simulink model "SMIB_test_SL_2023a_Copy"  (R2023a)
settings: Solver=FixedStepAuto  StartTime=0.0  StopTime=30.0  FixedStep=1e-4  RelTol=1e-3
undefined symbols (not defined in the file or in its folder): Angle, D1, Delta, Magnitude
libraries: spsThreePhaseSeriesRLCLoadLib x4, spsThreePhasePISectionLineLib x2, spsThreePhaseBreakerLib x2, ee_lib x1, spsExcitationSystemLib x1, spsHydraulicTurbineandGovernorLib x1, spsSynchronousMachinepuFundamentalLib x1, spsThreePhaseDynamicLoadLib x1, spsThreePhaseTransformerTwoWindingsLib x1, spsThreePhaseVIMeasurementLib x1, spsThreePhaseFaultLib x1, spsThreePhaseSourceLib x1
settings Model: Creator=shaohui  LastModifiedBy=lab-admin

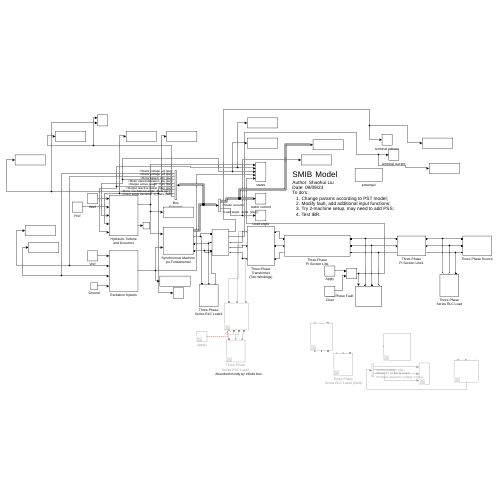
[thumbnail: Simulink's stored preview of the top-level diagram]
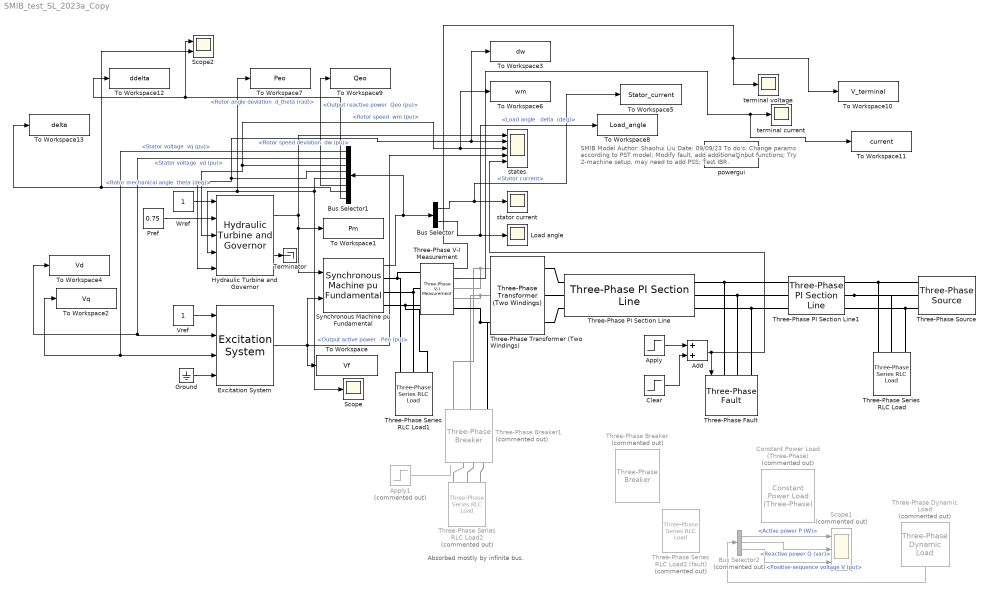
== system SMIB_test_SL_2023a_Copy ==
  note: Absorbed mostly by infinite bus.
  note: SMIB Model
      | Author: Shaohui Liu
      | Date: 09/09/23
      | To do's:
      | Change params according to PST model;
      | Modify fault, add additional input functions;
      | Try 2-machine setup, may need to add PSS;
      | Test IBR.
  Add : Sum
  Apply : Step  Time=15  After=5  SampleTime=0
  Apply1 : Step  Commented=on  Time=23  SampleTime=0
  Bus Selector : BusSelector  OutputSignals="Stator current,Load angle   delta  (deg)"
  Bus Selector1 : BusSelector  OutputSignals="dq0 components.Stator voltage  vq (pu),dq0 components.Stator voltage  vd (pu),Mechanical.Rotor speed  wm (pu),Mechanical.Rotor speed deviation  dw (pu),Output active power   Peo (pu),Output reactive power  Qeo (pu),Mechanical.Rotor mechanical angle  theta (deg),Mechanical.Rotor angle deviation  d_theta (rad)"
  Bus Selector2 : BusSelector  Commented=on  OutputSignals=Active power P (W),Reactive power Q (var),Positive-sequence voltage V (pu)
  Clear : Step  Time=15.1667  After=-5  SampleTime=0
  Constant Power Load (Three-Phase) : ee_lib/Passive/Constant Power Load (Three-Phase)  Commented=on  port_option=ee.enum.threePhasePort.composite  FRated=60 Hz  active_power=1 kW  reactive_power=0 A*kV  Vline_rms_min=100 V  tau=0.01 s  Vline_rms_ini=200 V  Vang_ini=0 deg  gmin=1e-6 S  enable_fault=simscape.enum.onoff.off  fault_action=simscape.enum.assert.action.none  t_fault=1 s  open_conductance=1e-4 S
      settings: InternalSimscapePortConfiguration="{\"Bottom\":[],\"Left\":[{\"id\":\"N\",\"label\":\"~\",\"type\":\"foundation.electrical.three_phase\"}],\"Right\":[],\"Top\":[]}"
  Excitation System : spsExcitationSystemLib/Excitation System  tr=20e-3  reg=[ 300, 0.001 ]  exc=[ 1, 0 ]  tgr=[ 0, 0 ]  damp=[ 0.001, 0.1 ]  sat=[ 0, 0 ]  lim=[ -11.5, 11.5, 0 ]  v0="[1.0  1.28]"
      settings: LibrarySourceBlock=sps_lib/Electrical Machines/Synchronous Machine Control/Excitation System
  Ground : Ground
  Hydraulic Turbine and Governor : spsHydraulicTurbineandGovernorLib/Hydraulic Turbine and Governor  sm="[ 10/3  0.07 ]"  gate="[  0.01  0.97518  -0.1  0.1 ]"  reg="[  0.05  1.163  0.105  0  0.01  ]"  hyd="[  0  2.67  ]"  dref=0  po=0.7516
      settings: LibrarySourceBlock=|
      | sps_lib/Electrical Machines/Synchronous Machine Control/Hydraulic Turbine
      | and Governor
  Load angle : Scope
  Pref : Constant  Value=0.75
  Scope : Scope
  Scope1 : Scope  Commented=on  NumInputPorts=3
  Scope2 : Scope  NumInputPorts=2
  Synchronous Machine pu Fundamental : spsSynchronousMachinepuFundamentalLib/Synchronous Machine pu Fundamental  PresetModel=No  MechanicalLoad=Mechanical power Pm  ShowDetailedParameters=on  RotorType=Salient-pole  Units=per unit fundamental parameters  MeasurementBus=off  NominalParameters="[ 187E6  13800   60]"  Stator="[ 2.85E-03  0.114  1.19  0.36 ]"  Field="[ 5.79E-04  0.114]"  Dampers2=[0.0652, 0.5134, 0.0287, 0.2553, 7.765e-3, 0.9167 ]  Dampers1="[ 1.17E-02  0.182  1.97E-02  0.384 ]"  Mechanical=[ 3.7 0 20]  PolePairs=20  InitialConditions="[ 0  0  0  0  0  0  0  0  1 ]"  SetSaturation=off  Saturation=[0.6404,0.7127,0.8441,0.9214,0.9956,1.082,1.19,1.316,1.457;0.7,0.7698,0.8872,0.9466,0.9969,1.046,1.1,1.151,1.201]  LoadFlowParameters=[1,0,0,0,0]  TsPowergui=0  TsBlock=-1  IterativeModel=Trapezoidal non iterative  IterativeDiscreteModel=Trapezoidal non iterative  BusType=PV  Pref=0  Qref=0  Qmin=-inf  Qmax=inf  PLF=0  QLF=0
      settings: LibrarySourceBlock=|
      | sps_lib/Electrical Machines/Synchronous Machine
      | pu Fundamental
  Terminator : Terminator
  Three-Phase Dynamic Load : spsThreePhaseDynamicLoadLib/Three-Phase Dynamic Load  Commented=on  NominalVoltage=[ 13.8e3 60 ]  ActiveReactivePowers=[50e6 25e6]  PositiveSequence=[0.994 -11.8]  ExternalControl=off  NpNq=[1.3 2]  TimeConstants="[0  0  0  0]"  MinimumVoltage=0.7  Tfilter=1e-4  LoadFlowParameters=[4,0,0,0,0]
      settings: LibrarySourceBlock=|
      | sps_lib/Passives/Three-Phase
      | Dynamic Load
  Three-Phase PI Section Line : spsThreePhasePISectionLineLib/Three-Phase PI Section Line  LConnTagsString=a|b|c  RConnTagsString=A|B|C  Length=95  Frequency=60  Resistances=[ 0.01273 0.3864]  Inductances="[ 0.9337e-3  4.1264e-3]"  Capacitances=[12.74e-9 7.751e-9]
  Three-Phase PI Section Line1 : spsThreePhasePISectionLineLib/Three-Phase PI Section Line  LConnTagsString=a|b|c  RConnTagsString=A|B|C  Length=5  Frequency=60  Resistances=[ 0.01273 0.3864]  Inductances="[ 0.9337e-3  4.1264e-3]"  Capacitances=[12.74e-9 7.751e-9]
  Three-Phase Series RLC Load : spsThreePhaseSeriesRLCLoadLib/Three-Phase Series RLC Load  LConnTagsString=A|B|C  Configuration=Y (grounded)  NominalVoltage=230e3  Vabc=[1e3 1e3 1e3]  Vabcp=[1e3 1e3 1e3]  NominalFrequency=60  UnbalancedPower=off  ActivePower=10e3  InductivePower=100  CapacitivePower=100  Pabc=[10e3 9e3 11e3]  QLabc=[100 90 110]  QCabc=[100 90 110]  Pabcp=[10e3 9e3 11e3]  QLabcp=[100 90 110]  QCabcp=[100 90 110]  Measurements=None  LoadType=constant Z
  Three-Phase Series RLC Load1 : spsThreePhaseSeriesRLCLoadLib/Three-Phase Series RLC Load  LConnTagsString=A|B|C  Configuration=Y (grounded)  NominalVoltage=13.8e3  Vabc=[1e3 1e3 1e3]  Vabcp=[1e3 1e3 1e3]  NominalFrequency=60  UnbalancedPower=off  ActivePower=10e3  InductivePower=0  CapacitivePower=0  Pabc=[10e3 9e3 11e3]  QLabc=[100 90 110]  QCabc=[100 90 110]  Pabcp=[10e3 9e3 11e3]  QLabcp=[100 90 110]  QCabcp=[100 90 110]  Measurements=None  LoadType=constant Z
  Three-Phase Series RLC Load2 : spsThreePhaseSeriesRLCLoadLib/Three-Phase Series RLC Load  Commented=on  LConnTagsString=A|B|C  Configuration=Y (grounded)  NominalVoltage=13.8e3  Vabc=[13.8e3 13.8e3 13.8e3]  Vabcp=[13.8e3 13.8e3 13.8e3]  NominalFrequency=60  UnbalancedPower=on  ActivePower=100e3  InductivePower=0  CapacitivePower=0  Pabc=[10000e3 10000e3 10000e3]  QLabc=[1000 1000 1000]  QCabc=[1000 1000 1000]  Pabcp=[1000e3 900e3 1100e3]  QLabcp=[100 90 110]  QCabcp=[100 90 110]  Measurements=None  LoadType=constant PQ
  Three-Phase Series RLC Load2 (fault) : spsThreePhaseSeriesRLCLoadLib/Three-Phase Series RLC Load  Commented=on  LConnTagsString=A|B|C  Configuration=Y (grounded)  NominalVoltage=13.8e3  Vabc=[1e3 1e3 1e3]  Vabcp=[1e3 1e3 1e3]  NominalFrequency=60  UnbalancedPower=off  ActivePower=100e3  InductivePower=100  CapacitivePower=100  Pabc=[10e3 9e3 11e3]  QLabc=[100 90 110]  QCabc=[100 90 110]  Pabcp=[10e3 9e3 11e3]  QLabcp=[100 90 110]  QCabcp=[100 90 110]  Measurements=Branch voltages and currents  LoadType=constant Z
  Three-Phase Transformer (Two Windings) : spsThreePhaseTransformerTwoWindingsLib/Three-Phase Transformer (Two Windings)  Winding1Connection=Delta (D1)  Winding2Connection=Yg  CoreType=Three single-phase transformers  SetSaturation=off  Hysteresis=off  DataFile='hysteresis'  SetInitialFlux=off  Measurements=None  UNITS=pu  NominalPower=[ 250e6 , 60 ]  Winding1=[13.8e3 , 0.002 , 0.08 ]  Winding2=[ 230e3 , 0.002 , 0.08 ]  Rm=500  Lm=500  L0=0.5  Saturation=[ 0,0 ; 0.0024,1.2 ; 1.0,1.52 ]  InitialFluxes=[ 0.8 , -0.8 , 0.7 ]  BreakLoop=off  DiscreteSolver=Trapezoidal iterative  DataType=off  TransfoNumber=1
  Three-Phase V-I Measurement : spsThreePhaseVIMeasurementLib/Three-Phase V-I Measurement  VoltageMeasurement=phase-to-phase  SetLabelV=off  LabelV=Vabc  Vpu=off  VpuLL=off  CurrentMeasurement=yes  SetLabelI=off  LabelI=Iabc  Ipu=off  Pbase=100e6  Vbase=500e3  OutputType=Magnitude-Angle  PhasorSimulation=on  PSBequivalent=0
  Three-Phase Breaker : spsThreePhaseBreakerLib/Three-Phase Breaker  Commented=on  InitialState=closed  SwitchA=on  SwitchB=on  SwitchC=on  SwitchTimes="[20.5  20.5+5/60]"  External=off  BreakerResistance=0.01  SnubberResistance=1e6  SnubberCapacitance=inf  Measurements=Breaker voltages and currents
  Three-Phase Breaker1 : spsThreePhaseBreakerLib/Three-Phase Breaker  Commented=on  InitialState=open  SwitchA=on  SwitchB=on  SwitchC=on  SwitchTimes="[23  23+30/60]"  External=on  BreakerResistance=0.01  SnubberResistance=1e6  SnubberCapacitance=inf  Measurements=None
  Three-Phase Fault : spsThreePhaseFaultLib/Three-Phase Fault  InitialStates=0  FaultA=on  FaultB=on  FaultC=on  GroundFault=on  SwitchTimes="[15  15+2/60]"  External=on  SwitchStatus=NaN  FaultResistance=0.001  GroundResistance=0.01  SnubberResistance=1e6  SnubberCapacitance=inf  Measurements=Fault voltages and currents
  Three-Phase Source : spsThreePhaseSourceLib/Three-Phase Source  InternalConnection=Yg  VoltagePhases=off  Voltage=230e3  PhaseAngle=0  Voltage_phases=[25e3 25e3 25e3]/sqrt(3)  PhaseAngles_phases=[0 -120 +120]  Frequency=60  NonIdealSource=on  SpecifyImpedance=off  Resistance=0.8929  Inductance=16.58e-3  ShortCircuitLevel=100e6  BaseVoltage=25e3  XRratio=7  BusType=swing  Pref=10e3  Qref=0  Prefabc=[10e3, 10e3, 10e3]  Qrefabc=[0, 0, 0]  Qmin=-inf  Qmax=inf
  To Workspace : ToWorkspace  VariableName=Vf  SaveFormat=Timeseries  SampleTime=-1
  To Workspace1 : ToWorkspace  VariableName=Pm  SaveFormat=Timeseries  SampleTime=-1
  To Workspace10 : ToWorkspace  VariableName=V_terminal  SaveFormat=Timeseries  SampleTime=-1
  To Workspace11 : ToWorkspace  VariableName=current  SaveFormat=Timeseries  SampleTime=-1
  To Workspace12 : ToWorkspace  VariableName=ddelta  SaveFormat=Timeseries  SampleTime=-1
  To Workspace13 : ToWorkspace  VariableName=delta  SaveFormat=Timeseries  SampleTime=-1
  To Workspace2 : ToWorkspace  VariableName=Vq  SaveFormat=Timeseries  SampleTime=-1
  To Workspace3 : ToWorkspace  VariableName=dw  SaveFormat=Timeseries  SampleTime=-1
  To Workspace4 : ToWorkspace  VariableName=Vd  SaveFormat=Timeseries  SampleTime=-1
  To Workspace5 : ToWorkspace  VariableName=Stator_current  SaveFormat=Timeseries  SampleTime=-1
  To Workspace6 : ToWorkspace  VariableName=wm  SaveFormat=Timeseries  SampleTime=-1
  To Workspace7 : ToWorkspace  VariableName=Peo  SaveFormat=Timeseries  SampleTime=-1
  To Workspace8 : ToWorkspace  VariableName=Load_angle  SaveFormat=Timeseries  SampleTime=-1
  To Workspace9 : ToWorkspace  VariableName=Qeo  SaveFormat=Timeseries  SampleTime=-1
  Vref : Constant
  Wref : Constant
  powergui : sps_lib/powergui  Priority=1  SimulationMode=Phasor  SampleTime=50e-6  frequency=60  Iterations=50  frequencyindice=60  Pbase=100e6  ErrMax=1e-4  UnitsV=kV  UnitsW=MW  buscounter=0  FunctionMessages=off  echomessages=off  EnableUseOfTLC=off  CurrentSourceSwitches=off  DisableSnubberDevices=off  DisableRonSwitches=off  DisableVfSwitches=off  DisplayEquations=off  AutomaticDiscreteSolvers=off  SolverType=Tustin/Backward Euler (TBE)  Interpol=off  ExternalGateDelay=off  methode=off  Ts=100  x0status=blocks  SPID=on  SwTol=0  HookPort=off  NonlinearTolerance=1e-4  nMaxIteration=100  ContinueOnMaxIteration=off  RestoreLinks=warning  ResistiveCurrentMeasurement=off  Frange=[0:2:500]  Ylog=off  Xlog=on  ShowGrid=off  save=off  variable=ZData  structure=0  ZoomFFT=off  StartTime=0.0  cycles=1  DisplayStyle=1  fundamental=60  FreqAxis=off  MaxFrequency=1000  frequencyindicesteady=1  RmsSteady=1  display=off
  states : Scope  NumInputPorts=5
  stator current : Scope
  terminal current : Scope
  terminal voltage : Scope
  wires:
  Hydraulic Turbine and Governor/1 -> To Workspace1/1, Synchronous Machine pu Fundamental/1, states/1
  Synchronous Machine pu Fundamental/1 -> Bus Selector1/1, Bus Selector/1
  Bus Selector/1 -> To Workspace5/1, stator current/1  "<Stator current>"
  Bus Selector/2 -> To Workspace8/1, Load angle/1  "<Load angle   delta  (deg)>"
  Wref/1 -> Hydraulic Turbine and Governor/1
  Pref/1 -> Hydraulic Turbine and Governor/2
  Bus Selector1/1 -> Excitation System/3, To Workspace2/1  "<Stator voltage  vq (pu)>"
  Bus Selector1/2 -> To Workspace4/1, Excitation System/2  "<Stator voltage  vd (pu)>"
  Bus Selector1/3 -> Hydraulic Turbine and Governor/3, To Workspace6/1, states/3  "<Rotor speed  wm (pu)>"
  Bus Selector1/4 -> Hydraulic Turbine and Governor/5, To Workspace3/1, states/2  "<Rotor speed deviation  dw (pu)>"
  Bus Selector1/5 -> To Workspace7/1, Hydraulic Turbine and Governor/4, Scope/1  "<Output active power   Peo (pu)>"
  Vref/1 -> Excitation System/1
  Ground/1 -> Excitation System/4
  Hydraulic Turbine and Governor/2 -> Terminator/1
  Add/1 -> states/5, Three-Phase Fault/1
  Apply/1 -> Add/1
  Clear/1 -> Add/2
  Apply1/1 -> ?
  Three-Phase Dynamic Load/1 -> Bus Selector2/1
  Bus Selector2/1 -> Scope1/1  "<Active power P (W)>"
  Bus Selector2/2 -> Scope1/2  "<Reactive power Q (var)>"
  Bus Selector2/3 -> Scope1/3  "<Positive-sequence voltage V (pu)>"
  Excitation System/1 -> To Workspace/1, states/4, Synchronous Machine pu Fundamental/2
  Bus Selector1/6 -> To Workspace9/1  "<Output reactive power  Qeo (pu)>"
  Three-Phase V-I Measurement/1 -> To Workspace10/1, terminal voltage/1
  Three-Phase V-I Measurement/2 -> To Workspace11/1, terminal current/1
  Bus Selector1/7 -> To Workspace13/1, Scope2/2  "<Rotor mechanical angle  theta (deg)>"
  Bus Selector1/8 -> Scope2/1, To Workspace12/1  "<Rotor angle deviation  d_theta (rad)>"
  connections:
  Three-Phase Breaker1/RConn1 -- Three-Phase V-I Measurement/RConn1 -- Three-Phase Transformer (Two Windings)/LConn1
  Three-Phase Breaker1/RConn2 -- Three-Phase V-I Measurement/RConn2 -- Three-Phase Transformer (Two Windings)/LConn2
  Three-Phase Transformer (Two Windings)/RConn1 -- Three-Phase PI Section Line/LConn1
  Three-Phase Transformer (Two Windings)/RConn2 -- Three-Phase PI Section Line/LConn2
  Three-Phase Transformer (Two Windings)/RConn3 -- Three-Phase PI Section Line/LConn3
  Three-Phase Series RLC Load/LConn1 -- Three-Phase Source/RConn1 -- Three-Phase PI Section Line1/RConn1
  Three-Phase PI Section Line/RConn2 -- Three-Phase Fault/LConn2 -- Three-Phase PI Section Line1/LConn2
  Three-Phase Series RLC Load/LConn3 -- Three-Phase PI Section Line1/RConn3 -- Three-Phase Source/RConn3
  Three-Phase Series RLC Load2/LConn1 -- Three-Phase Breaker1/LConn1
  Three-Phase Series RLC Load2/LConn2 -- Three-Phase Breaker1/LConn2
  Three-Phase Series RLC Load2/LConn3 -- Three-Phase Breaker1/LConn3
  Three-Phase PI Section Line/RConn3 -- Three-Phase PI Section Line1/LConn3 -- Three-Phase Fault/LConn3
  Three-Phase PI Section Line1/RConn2 -- Three-Phase Source/RConn2 -- Three-Phase Series RLC Load/LConn2
  Three-Phase PI Section Line1/LConn1 -- Three-Phase PI Section Line/RConn1 -- Three-Phase Fault/LConn1
  Three-Phase Series RLC Load1/LConn1 -- Three-Phase V-I Measurement/LConn1 -- Synchronous Machine pu Fundamental/RConn1
  Three-Phase Series RLC Load1/LConn2 -- Three-Phase V-I Measurement/LConn2 -- Synchronous Machine pu Fundamental/RConn2
  Three-Phase Series RLC Load1/LConn3 -- Synchronous Machine pu Fundamental/RConn3 -- Three-Phase V-I Measurement/LConn3
  Three-Phase Transformer (Two Windings)/LConn3 -- Three-Phase Breaker1/RConn3 -- Three-Phase V-I Measurement/RConn3
